simulink model "ModeState32Bit"  (R2018b)
settings: Solver=FixedStepDiscrete  StartTime=0.0  StopTime=10.0  FixedStep=0.01  RelTol=1e-3
settings Model: Creator=sn2xws  LastModifiedBy=sn2xws
settings DataIOCC: SaveFormat=StructureWithTime
settings OptimizationCC: DefaultParameterBehavior=Inlined  EnhancedBackFolding=on  PassReuseOutputArgsAs=Individual arguments  ZeroExternalMemoryAtStartup=off  ZeroInternalMemoryAtStartup=off  OptimizeBlockOrder=speed  DifferentSizesBufferReuse=on  OptimizationCustomize=off
settings DebuggingCC: ParameterTunabilityLossMsg=error
settings ModelReferenceCC: ModelReferenceNumInstancesAllowed=Single
settings SFSimCC: MATLABDynamicMemAlloc=off
settings RTWCC: SystemTargetFile=autosar.tlc  GenCodeOnly=on  TemplateMakefile=ert_default_tmf  Description=AUTOSAR  GenerateReport=on  IncludeHyperlinkInReport=on  LaunchReport=on  GenerateTraceInfo=on  GenerateTraceReport=on  GenerateTraceReportSl=on  GenerateTraceReportSf=on  GenerateTraceReportEml=on
settings CodeAppCC: ForceParamTrailComments=on  IgnoreCustomStorageClasses=off  OperatorAnnotations=on  SimulinkDataObjDesc=on  SFDataObjDesc=on  InsertBlockDesc=on
settings STFCustomTargetCC: TargetLangStandard=C99 (ISO)  MultiwordLength=256  ParMdlRefBuildCompliant=on  CompOptLevelCompliant=on  IncludeMdlTerminateFcn=off  CombineOutputUpdateFcns=on  SuppressErrorStatus=on  ERTCustomFileBanners=on  SupportNonFinite=off  SupportComplex=off  SupportContinuousTime=off  SupportNonInlinedSFcns=off  RemoveResetFunc=on  MATLABClassNameForMDSCustomization=Simulink.SoftwareTarget.ERTCustomization  AutosarCompliant=on  UseToolchainInfoCompliant=on  LookupTableObjectStructAxisOrder=2,1,3,4,...  LUTObjectStructOrderEvenSpacing=Size,Table,Breakpoints  SystemTargetFile=autosar.tlc
settings ERTTargetCC: TargetLangStandard=C99 (ISO)  ConcurrentExecutionCompliant=off  IncludeMdlTerminateFcn=off  SuppressErrorStatus=on  SupportNonFinite=off  SupportComplex=off  ModelStepFunctionPrototypeControlCompliant=off  CPPClassGenCompliant=off  AutosarCompliant=on  LookupTableObjectStructAxisOrder=2,1,3,4,...  LUTObjectStructOrderEvenSpacing=Size,Table,Breakpoints  InlinedParameterPlacement=NonHierarchical  ERTCustomFileTemplate=example_file_process.tlc

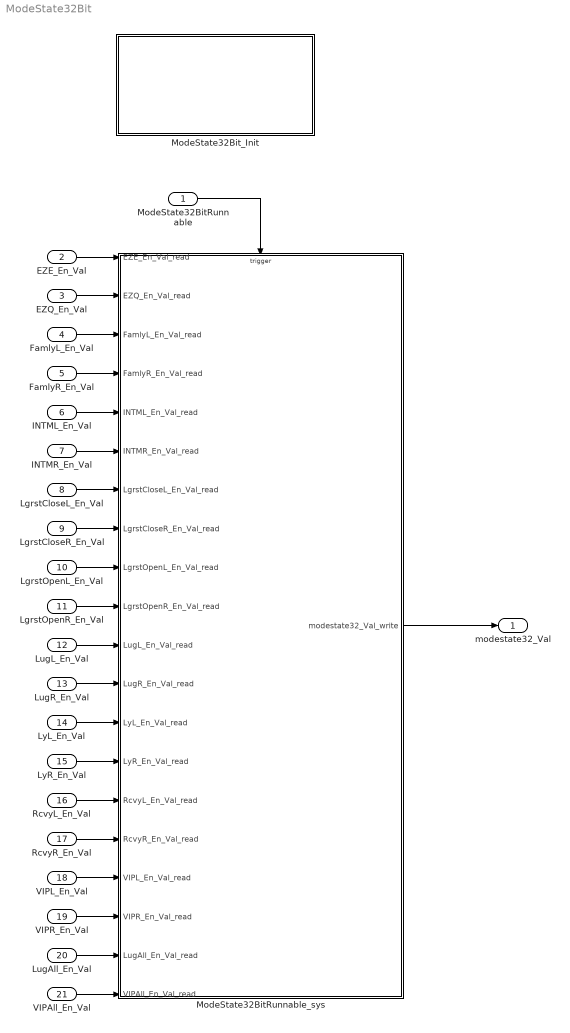
== system ModeState32Bit ==
  ModeState32BitRunnable : Inport  SampleTime=0.01  OutputFunctionCall=on
  EZE_En_Val : Inport  Port=2  OutDataTypeStr=boolean  PortDimensions=1
  EZQ_En_Val : Inport  Port=3  OutDataTypeStr=boolean  PortDimensions=1
  FamlyL_En_Val : Inport  Port=4  OutDataTypeStr=boolean  PortDimensions=1
  FamlyR_En_Val : Inport  Port=5  OutDataTypeStr=boolean  PortDimensions=1
  INTML_En_Val : Inport  Port=6  OutDataTypeStr=boolean  PortDimensions=1
  INTMR_En_Val : Inport  Port=7  OutDataTypeStr=boolean  PortDimensions=1
  LgrstCloseL_En_Val : Inport  Port=8  OutDataTypeStr=boolean  PortDimensions=1
  LgrstCloseR_En_Val : Inport  Port=9  OutDataTypeStr=boolean  PortDimensions=1
  LgrstOpenL_En_Val : Inport  Port=10  OutDataTypeStr=boolean  PortDimensions=1
  LgrstOpenR_En_Val : Inport  Port=11  OutDataTypeStr=boolean  PortDimensions=1
  LugL_En_Val : Inport  Port=12  OutDataTypeStr=boolean  PortDimensions=1
  LugR_En_Val : Inport  Port=13  OutDataTypeStr=boolean  PortDimensions=1
  LyL_En_Val : Inport  Port=14  OutDataTypeStr=boolean  PortDimensions=1
  LyR_En_Val : Inport  Port=15  OutDataTypeStr=boolean  PortDimensions=1
  RcvyL_En_Val : Inport  Port=16  OutDataTypeStr=boolean  PortDimensions=1
  RcvyR_En_Val : Inport  Port=17  OutDataTypeStr=boolean  PortDimensions=1
  VIPL_En_Val : Inport  Port=18  OutDataTypeStr=boolean  PortDimensions=1
  VIPR_En_Val : Inport  Port=19  OutDataTypeStr=boolean  PortDimensions=1
  LugAll_En_Val : Inport  Port=20  OutDataTypeStr=boolean  PortDimensions=1
  VIPAll_En_Val : Inport  Port=21  OutDataTypeStr=boolean  PortDimensions=1
  ModeState32BitRunnable_sys : Subsystem
  ModeState32Bit_Init : Subsystem
  modestate32_Val : Outport  OutDataTypeStr=uint32  PortDimensions=1
  wires:
  EZE_En_Val/1 -> ModeState32BitRunnable_sys/1(EZE_En_Val_read)
  EZQ_En_Val/1 -> ModeState32BitRunnable_sys/2(EZQ_En_Val_read)
  FamlyL_En_Val/1 -> ModeState32BitRunnable_sys/3(FamlyL_En_Val_read)
  FamlyR_En_Val/1 -> ModeState32BitRunnable_sys/4(FamlyR_En_Val_read)
  INTML_En_Val/1 -> ModeState32BitRunnable_sys/5(INTML_En_Val_read)
  INTMR_En_Val/1 -> ModeState32BitRunnable_sys/6(INTMR_En_Val_read)
  LgrstCloseL_En_Val/1 -> ModeState32BitRunnable_sys/7(LgrstCloseL_En_Val_read)
  LgrstCloseR_En_Val/1 -> ModeState32BitRunnable_sys/8(LgrstCloseR_En_Val_read)
  LgrstOpenL_En_Val/1 -> ModeState32BitRunnable_sys/9(LgrstOpenL_En_Val_read)
  LgrstOpenR_En_Val/1 -> ModeState32BitRunnable_sys/10(LgrstOpenR_En_Val_read)
  LugL_En_Val/1 -> ModeState32BitRunnable_sys/11(LugL_En_Val_read)
  LugR_En_Val/1 -> ModeState32BitRunnable_sys/12(LugR_En_Val_read)
  LyL_En_Val/1 -> ModeState32BitRunnable_sys/13(LyL_En_Val_read)
  LyR_En_Val/1 -> ModeState32BitRunnable_sys/14(LyR_En_Val_read)
  RcvyL_En_Val/1 -> ModeState32BitRunnable_sys/15(RcvyL_En_Val_read)
  RcvyR_En_Val/1 -> ModeState32BitRunnable_sys/16(RcvyR_En_Val_read)
  VIPL_En_Val/1 -> ModeState32BitRunnable_sys/17(VIPL_En_Val_read)
  VIPR_En_Val/1 -> ModeState32BitRunnable_sys/18(VIPR_En_Val_read)
  ModeState32BitRunnable_sys/1(modestate32_Val_write) -> modestate32_Val/1
  ModeState32BitRunnable/1 -> ModeState32BitRunnable_sys/Trigger
  LugAll_En_Val/1 -> ModeState32BitRunnable_sys/19(LugAll_En_Val_read)
  VIPAll_En_Val/1 -> ModeState32BitRunnable_sys/20(VIPAll_En_Val_read)

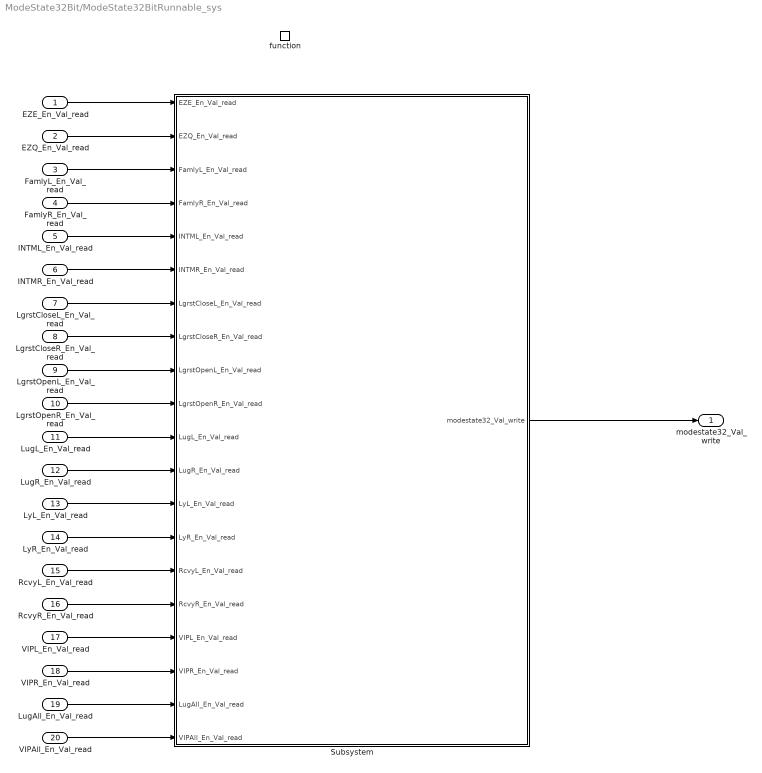
== system ModeState32Bit/ModeState32BitRunnable_sys ==
  EZE_En_Val_read : Inport
  EZQ_En_Val_read : Inport  Port=2
  FamlyL_En_Val_read : Inport  Port=3
  FamlyR_En_Val_read : Inport  Port=4
  INTML_En_Val_read : Inport  Port=5
  INTMR_En_Val_read : Inport  Port=6
  LgrstCloseL_En_Val_read : Inport  Port=7
  LgrstCloseR_En_Val_read : Inport  Port=8
  LgrstOpenL_En_Val_read : Inport  Port=9
  LgrstOpenR_En_Val_read : Inport  Port=10
  LugL_En_Val_read : Inport  Port=11
  LugR_En_Val_read : Inport  Port=12
  LyL_En_Val_read : Inport  Port=13
  LyR_En_Val_read : Inport  Port=14
  RcvyL_En_Val_read : Inport  Port=15
  RcvyR_En_Val_read : Inport  Port=16
  VIPL_En_Val_read : Inport  Port=17
  VIPR_En_Val_read : Inport  Port=18
  LugAll_En_Val_read : Inport  Port=19
  VIPAll_En_Val_read : Inport  Port=20
  function : TriggerPort  TriggerType=function-call  VariantControl=(inherit)  SampleTimeType=periodic  SampleTime=-1
  Subsystem : Subsystem
  modestate32_Val_write : Outport
      settings: EnsureOutportIsVirtual=on
  wires:
  EZE_En_Val_read/1 -> Subsystem/1(EZE_En_Val_read)
  EZQ_En_Val_read/1 -> Subsystem/2(EZQ_En_Val_read)
  FamlyL_En_Val_read/1 -> Subsystem/3(FamlyL_En_Val_read)
  FamlyR_En_Val_read/1 -> Subsystem/4(FamlyR_En_Val_read)
  INTML_En_Val_read/1 -> Subsystem/5(INTML_En_Val_read)
  INTMR_En_Val_read/1 -> Subsystem/6(INTMR_En_Val_read)
  LgrstCloseL_En_Val_read/1 -> Subsystem/7(LgrstCloseL_En_Val_read)
  LgrstCloseR_En_Val_read/1 -> Subsystem/8(LgrstCloseR_En_Val_read)
  LgrstOpenL_En_Val_read/1 -> Subsystem/9(LgrstOpenL_En_Val_read)
  LgrstOpenR_En_Val_read/1 -> Subsystem/10(LgrstOpenR_En_Val_read)
  LugL_En_Val_read/1 -> Subsystem/11(LugL_En_Val_read)
  LugR_En_Val_read/1 -> Subsystem/12(LugR_En_Val_read)
  LyL_En_Val_read/1 -> Subsystem/13(LyL_En_Val_read)
  LyR_En_Val_read/1 -> Subsystem/14(LyR_En_Val_read)
  RcvyL_En_Val_read/1 -> Subsystem/15(RcvyL_En_Val_read)
  RcvyR_En_Val_read/1 -> Subsystem/16(RcvyR_En_Val_read)
  VIPL_En_Val_read/1 -> Subsystem/17(VIPL_En_Val_read)
  VIPR_En_Val_read/1 -> Subsystem/18(VIPR_En_Val_read)
  Subsystem/1(modestate32_Val_write) -> modestate32_Val_write/1
  LugAll_En_Val_read/1 -> Subsystem/19(LugAll_En_Val_read)
  VIPAll_En_Val_read/1 -> Subsystem/20(VIPAll_En_Val_read)

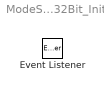
== system ModeState32Bit/ModeState32Bit_Init ==
  Event Listener : EventListener  EventName=reset

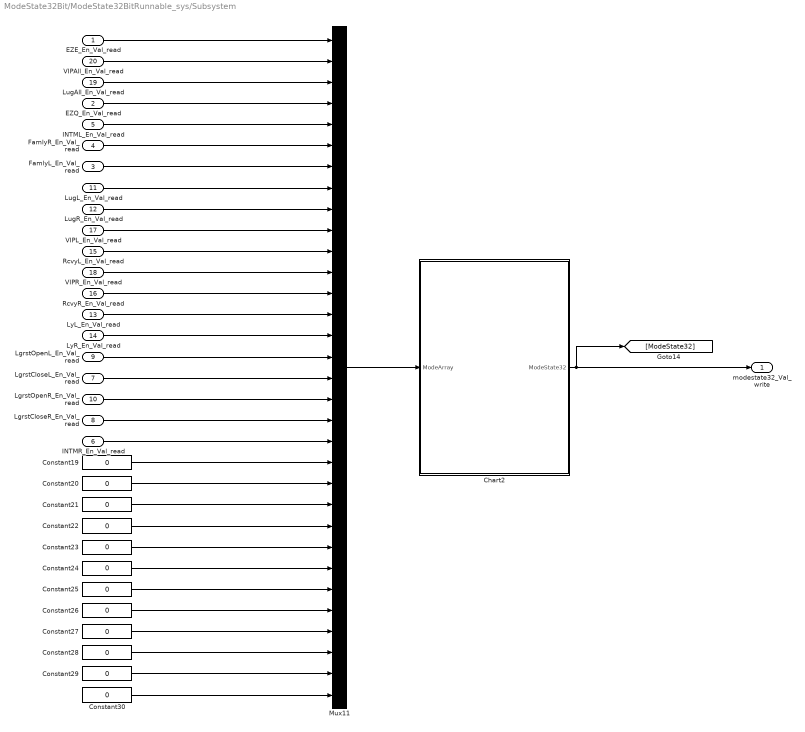
== system ModeState32Bit/ModeState32BitRunnable_sys/Subsystem ==
  EZE_En_Val_read : Inport
  EZQ_En_Val_read : Inport  Port=2
  FamlyL_En_Val_read : Inport  Port=3
  FamlyR_En_Val_read : Inport  Port=4
  INTML_En_Val_read : Inport  Port=5
  INTMR_En_Val_read : Inport  Port=6
  LgrstCloseL_En_Val_read : Inport  Port=7
  LgrstCloseR_En_Val_read : Inport  Port=8
  LgrstOpenL_En_Val_read : Inport  Port=9
  LgrstOpenR_En_Val_read : Inport  Port=10
  LugL_En_Val_read : Inport  Port=11
  LugR_En_Val_read : Inport  Port=12
  LyL_En_Val_read : Inport  Port=13
  LyR_En_Val_read : Inport  Port=14
  RcvyL_En_Val_read : Inport  Port=15
  RcvyR_En_Val_read : Inport  Port=16
  VIPL_En_Val_read : Inport  Port=17
  VIPR_En_Val_read : Inport  Port=18
  LugAll_En_Val_read : Inport  Port=19
  VIPAll_En_Val_read : Inport  Port=20
  Chart2 : Stateflow chart  TreatAsAtomicUnit=on
  Constant{19..30} (12 alike) : Constant  Description=_SGMK226P2.FCMD.000_369_  Value=0  OutDataTypeStr=boolean
  Mux11 : Mux  Inputs=32
  modestate32_Val_write : Outport
      settings: EnsureOutportIsVirtual=on
  wires:
  EZE_En_Val_read/1 -> Mux11/1
  Mux11/1 -> Chart2/1(ModeArray)
  Constant20/1 -> Mux11/22
  FamlyR_En_Val_read/1 -> Mux11/6
  Constant30/1 -> Mux11/32
  Constant29/1 -> Mux11/31
  Constant27/1 -> Mux11/29
  LugL_En_Val_read/1 -> Mux11/8
  Constant25/1 -> Mux11/27
  LyL_En_Val_read/1 -> Mux11/14
  Constant19/1 -> Mux11/21
  Constant22/1 -> Mux11/24
  VIPAll_En_Val_read/1 -> Mux11/2
  LgrstOpenL_En_Val_read/1 -> Mux11/16
  EZQ_En_Val_read/1 -> Mux11/4
  INTML_En_Val_read/1 -> Mux11/5
  Constant21/1 -> Mux11/23
  Constant28/1 -> Mux11/30
  LgrstOpenR_En_Val_read/1 -> Mux11/18
  Chart2/1(ModeState32) -> [ModeState32], modestate32_Val_write/1
  LugAll_En_Val_read/1 -> Mux11/3
  FamlyL_En_Val_read/1 -> Mux11/7
  Constant23/1 -> Mux11/25
  VIPL_En_Val_read/1 -> Mux11/10
  LugR_En_Val_read/1 -> Mux11/9
  VIPR_En_Val_read/1 -> Mux11/12
  LyR_En_Val_read/1 -> Mux11/15
  RcvyR_En_Val_read/1 -> Mux11/13
  Constant24/1 -> Mux11/26
  RcvyL_En_Val_read/1 -> Mux11/11
  LgrstCloseL_En_Val_read/1 -> Mux11/17
  INTMR_En_Val_read/1 -> Mux11/20
  Constant26/1 -> Mux11/28
  LgrstCloseR_En_Val_read/1 -> Mux11/19

== stateflow chart ModeState32Bit/ModeState32BitRunnable_sys/Subsystem/Chart2 ==
  (default) -> (junction 3) : {ModeState32 = 0x00000000;}
  (junction 3) -> (junction 9) : {i = 0;}
  (junction 9) -> (junction 4) [order 1] : [i < 32]
  (junction 4) -> (junction 1) : {
      | temp_var = uint32(ModeArray[i]);
      | temp_var= temp_var << i;
      | ModeState32 = ModeState32 |  temp_var;
      | }
  (junction 1) -> (junction 9) : {i++;}
  (junction 9) -> (junction 5) [order 2]
  data: ModeState32 output uint32; ModeArray input boolean size=32; temp_var local uint32; i local uint8
